simulink model "QAM2016"  (R2016a)
settings: Solver=FixedStepDiscrete  StartTime=0.0  StopTime=0.2  FixedStep=1/2000000  RelTol=1e-3
libraries: dsparch4 x8
settings Model: Creator=beac2832  LastModifiedBy=beac2832
settings SolverCC: AutoInsertRateTranBlk=on

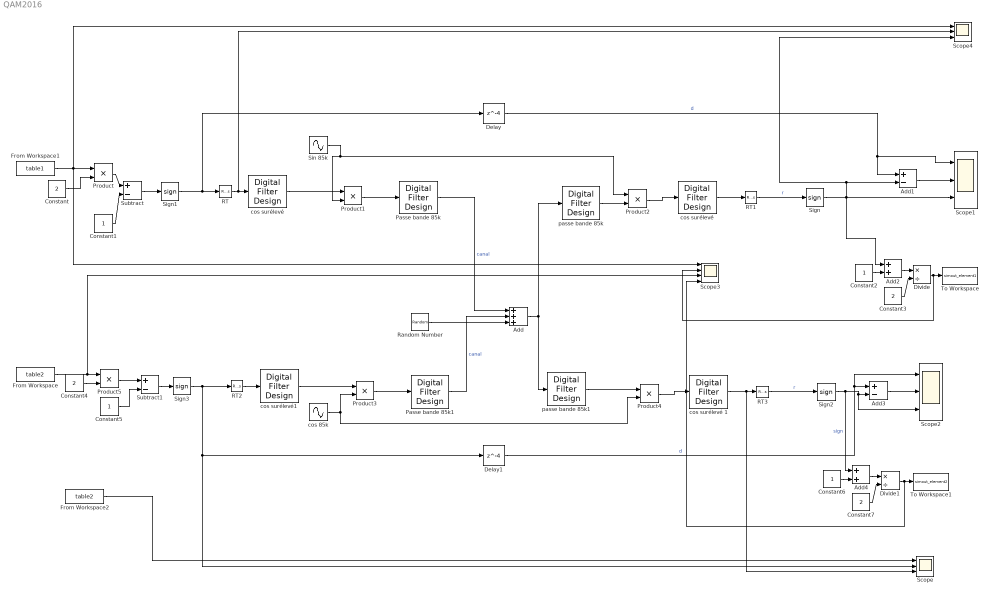
== system QAM2016 ==
  Add : Sum  Inputs=+++
  Add1 : Sum  Inputs=+-
  Add2 : Sum
  Add3 : Sum  Inputs=+-
  Add4 : Sum
  Constant{,3..4,7} (4 alike) : Constant  Value=2
  Constant{1..2,5..6} (4 alike) : Constant
  Delay : Delay  DelayLength=4  InitialCondition=0
  Delay1 : Delay  DelayLength=4  InitialCondition=0
  Divide : Product  Inputs=*/
  Divide1 : Product  Inputs=*/
  From Workspace : FromWorkspace  VariableName=table2
  From Workspace1 : FromWorkspace  VariableName=table1
  From Workspace2 : FromWorkspace  VariableName=table2  SampleTime=0
  Passe bande 85k : dsparch4/Digital Filter Design  mwdsp_browser_bugfix_var=off
  Passe bande 85k1 : dsparch4/Digital Filter Design  mwdsp_browser_bugfix_var=off
  Product{,1..5} (6 alike) : Product
  RT : RateTransition  OutPortSampleTime=5e-07
  RT1 : RateTransition  OutPortSampleTime=1/1000
  RT2 : RateTransition  OutPortSampleTime=5e-07
  RT3 : RateTransition  OutPortSampleTime=1/1000
  Random Number : RandomNumber  Variance=5  SampleTime=1/2000000
  Scope{,1..2,4} (4 alike) : Scope  NumInputPorts=3
  Scope3 : Scope  NumInputPorts=4
  Sign{,1..3} (4 alike) : Signum
  Sin 85k : Sin  Frequency=85000*2*pi  SampleTime=1/2000000
  Subtract : Sum  Inputs=+-
  Subtract1 : Sum  Inputs=+-
  To Workspace : ToWorkspace  VariableName=simout_element1  SaveFormat=Structure With Time  SampleTime=1/1000
      settings: Save2DSignal=2-D array (concatenate along first dimension)
  To Workspace1 : ToWorkspace  VariableName=simout_element2  SaveFormat=Structure With Time  SampleTime=-1
      settings: Save2DSignal=2-D array (concatenate along first dimension)
  cos 85k : Sin  Frequency=85000*2*pi  Phase=pi/2  SampleTime=1/2000000
  cos surélevé : dsparch4/Digital Filter Design  mwdsp_browser_bugfix_var=off
  "cos surélevé " : dsparch4/Digital Filter Design  mwdsp_browser_bugfix_var=off
  cos surélevé 1 : dsparch4/Digital Filter Design  mwdsp_browser_bugfix_var=off
  cos surélevé1 : dsparch4/Digital Filter Design  mwdsp_browser_bugfix_var=off
  passe bande 85k : dsparch4/Digital Filter Design  mwdsp_browser_bugfix_var=off
  passe bande 85k1 : dsparch4/Digital Filter Design  mwdsp_browser_bugfix_var=off
  wires:
  Product1/1 -> Passe bande 85k/1
  Product2/1 -> "cos surélevé "/1
  Delay/1 -> Scope1/1, Add1/1  "d"
  Sign1/1 -> Delay/1, RT/1
  cos surélevé/1 -> Product1/1
  Sin 85k/1 -> Product2/1, Product1/2
  Passe bande 85k/1 -> Add/1  "canal"
  RT1/1 -> Sign/1  "r"
  Add1/1 -> Scope1/2
  Add/1 -> passe bande 85k1/1, passe bande 85k/1
  "cos surélevé "/1 -> RT1/1
  Product3/1 -> Passe bande 85k1/1
  Product4/1 -> cos surélevé 1/1
  Delay1/1 -> Scope2/1, Add3/1  "d"
  RT2/1 -> cos surélevé1/1
  Sign3/1 -> Scope/2, Delay1/1, RT2/1
  cos surélevé1/1 -> Product3/1
  cos 85k/1 -> Product3/2, Product4/2
  Passe bande 85k1/1 -> Add/2  "canal"
  RT3/1 -> Sign2/1  "r"
  Add3/1 -> Scope2/2
  cos surélevé 1/1 -> Scope/3, RT3/1
  Sign2/1 -> Add4/1, Scope2/3, Add3/2  "sign"
  Random Number/1 -> Add/3
  From Workspace1/1 -> Scope4/1, Scope3/1, Product/1
  Product/1 -> Subtract/1
  Constant1/1 -> Subtract/2
  Constant/1 -> Product/2
  Subtract/1 -> Sign1/1
  Add2/1 -> Divide/1
  Divide/1 -> Scope3/2, To Workspace/1
  Constant3/1 -> Divide/2
  Constant2/1 -> Add2/2
  From Workspace/1 -> Scope3/3, Product5/1
  Product5/1 -> Subtract1/1
  Constant5/1 -> Subtract1/2
  Constant4/1 -> Product5/2
  Subtract1/1 -> Sign3/1
  Add4/1 -> Divide1/1
  Constant7/1 -> Divide1/2
  Constant6/1 -> Add4/2
  Divide1/1 -> Scope3/4, To Workspace1/1
  passe bande 85k1/1 -> Product4/1
  passe bande 85k/1 -> Product2/2
  From Workspace2/1 -> Scope/1
  Sign/1 -> Scope4/3, Add1/2, Add2/1, Scope1/3
  RT/1 -> Scope4/2, cos surélevé/1
